simulink model "test"  (R2020a)
settings: Solver=FixedStepAuto  StartTime=0.0  StopTime=10.0  FixedStep=1e-3  RelTol=1e-3  EnableMultiTasking=on
libraries: frdmk64flib x5, etargetslib x2
settings Model: ExtModeTrigDuration=5  Creator=Windows  LastModifiedBy=Max
settings OptimizationCC: EnhancedBackFolding=on  PassReuseOutputArgsAs=Individual arguments  ZeroExternalMemoryAtStartup=off  ZeroInternalMemoryAtStartup=off  MaxStackSize=64  OptimizeBlockOrder=speed  DifferentSizesBufferReuse=on  OptimizationCustomize=off  EfficientTunableParamExpr=on
settings DebuggingCC: ParameterTunabilityLossMsg=error
settings HardwareCC: ProdBitPerPointer=32  ProdBitPerSizeT=32  ProdBitPerPtrDiffT=32  ProdLargestAtomicInteger=Long  ProdLargestAtomicFloat=Double  ProdWordSize=32  ProdHWDeviceType=ARM Compatible->ARM Cortex
settings SFSimCC: MATLABDynamicMemAlloc=off
settings RTWCC: SystemTargetFile=ert.tlc  HardwareBoard=NXP FRDM-K64F  TemplateMakefile=ert_default_tmf  Toolchain=GNU Tools for ARM Embedded Processors
settings CodeAppCC: ForceParamTrailComments=on  IgnoreCustomStorageClasses=off  OperatorAnnotations=on  SimulinkDataObjDesc=on  SFDataObjDesc=on  InsertBlockDesc=on

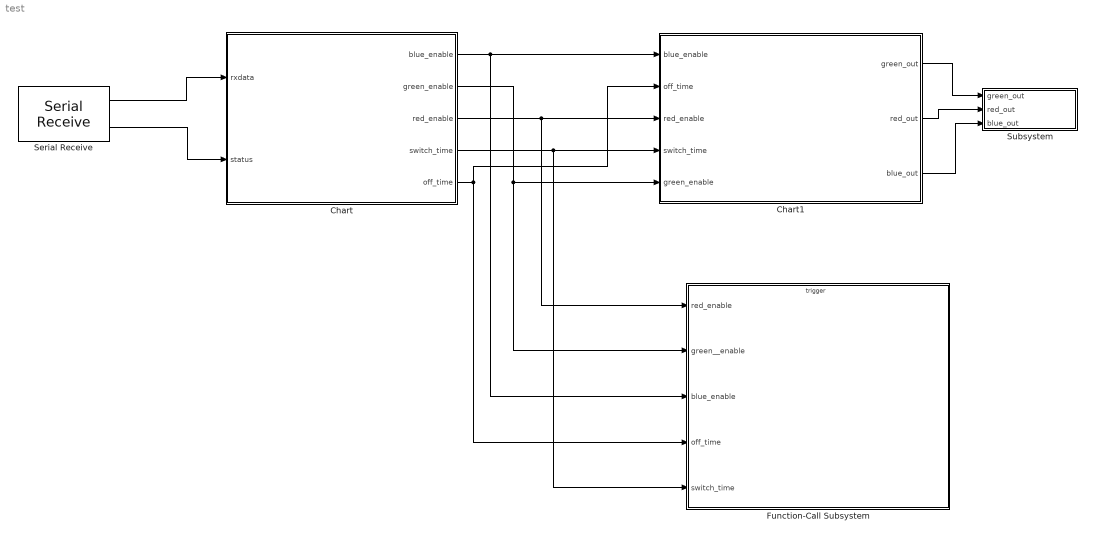
== system test ==
  Chart : Stateflow chart  TreatAsAtomicUnit=on
  Chart1 : Stateflow chart  TreatAsAtomicUnit=on
  Function-Call Subsystem : Subsystem  TreatAsAtomicUnit=on
  Serial Receive : frdmk64flib/Serial Receive  SCIModule=0  Baudrate=uint32(9600)  Parity=None  StopBits=1  HardwareFlowControl=None  ByteOrder=LittleEndian  DataType=uint8  DataLength=11  BlockingMode=off  OutputStatus=on  SampleTime=-1
  Subsystem : Subsystem
  wires:
  Serial Receive/1 -> Chart/1(rxdata)
  Serial Receive/2 -> Chart/2(status)
  Chart1/3(blue_out) -> Subsystem/3(blue_out)
  Chart/5(off_time) -> Function-Call Subsystem/4(off_time), Chart1/2(off_time)
  Chart/4(switch_time) -> Function-Call Subsystem/5(switch_time), Chart1/4(switch_time)
  Chart/3(red_enable) -> Function-Call Subsystem/1(red_enable), Chart1/3(red_enable)
  Chart/2(green_enable) -> Function-Call Subsystem/2(green__enable), Chart1/5(green_enable)
  Chart/1(blue_enable) -> Function-Call Subsystem/3(blue_enable), Chart1/1(blue_enable)
  Chart1/2(red_out) -> Subsystem/2(red_out)
  Chart1/1(green_out) -> Subsystem/1(green_out)

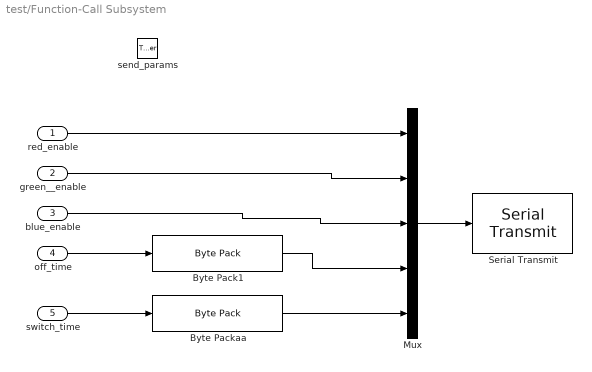
== system test/Function-Call Subsystem ==
  red_enable : Inport
  green__enable : Inport  Port=2
  blue_enable : Inport  Port=3
  off_time : Inport  Port=4
  switch_time : Inport  Port=5
  send_params : TriggerPort  TriggerType=function-call  IsSimulinkFunction=on  FunctionName=send_params  VariantControl=Variant
  Byte Pack1 : etargetslib/Byte Pack  datatypes={'single'}  byteAlign=1
  Byte Packaa : etargetslib/Byte Pack  datatypes={'uint16'}  byteAlign=1
  Mux : Mux  Inputs=5
  Serial Transmit : frdmk64flib/Serial Transmit  SCIModule=0  Baudrate=uint32(9600)  Parity=None  StopBits=1  HardwareFlowControl=None  ByteOrder=LittleEndian  BlockingMode=on  OutputStatus=off
  wires:
  red_enable/1 -> Mux/1
  switch_time/1 -> Byte Packaa/1
  off_time/1 -> Byte Pack1/1
  green__enable/1 -> Mux/2
  blue_enable/1 -> Mux/3
  Byte Pack1/1 -> Mux/4
  Byte Packaa/1 -> Mux/5
  Mux/1 -> Serial Transmit/1

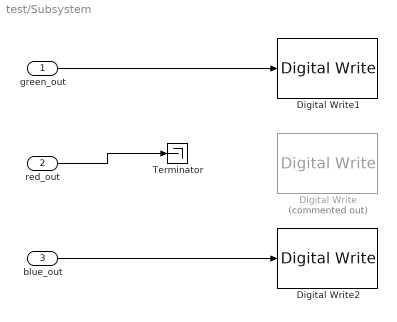
== system test/Subsystem ==
  green_out : Inport
  red_out : Inport  Port=2  OutDataTypeStr=boolean
  blue_out : Inport  Port=3
  Digital Write : frdmk64flib/Digital Write  Commented=on  Whichpin=RED_LED
  Digital Write1 : frdmk64flib/Digital Write  Whichpin=GREEN_LED
  Digital Write2 : frdmk64flib/Digital Write  Whichpin=BLUE_LED
  Terminator : Terminator
  wires:
  green_out/1 -> Digital Write1/1
  blue_out/1 -> Digital Write2/1
  red_out/1 -> Terminator/1

== stateflow chart test/Chart1 ==
  state OFF
    entry:
    red_out=false;
    green_out=false;
    blue_out=false;
  state RED_ON
    entry:
    red_out=true;
    green_out=false;
    blue_out=false;
  state BLUE_ON
    entry:
    red_out=false;
    green_out=false;
    blue_out=true;
  state GREEN_ON
    entry:
    red_out=false;
    green_out=true;
    blue_out=false;
  note: after(switch_time, msec)
  (default) -> OFF
  OFF -> (junction 3) : after(off_time, sec)
  (junction 3) -> RED_ON [order 1] : [red_enable==1]
  (junction 3) -> (junction 5) [order 2]
  RED_ON -> (junction 5) : after(switch_time,msec)
  (junction 4) -> OFF
  (junction 8) -> (junction 4) [order 2]
  (junction 5) -> (junction 8) [order 2]
  BLUE_ON -> (junction 4) : after(switch_time, msec)
  (junction 5) -> GREEN_ON [order 1] : [green_enable==1]
  (junction 8) -> BLUE_ON [order 1] : [blue_enable==1]
  GREEN_ON -> (junction 8)
  data: blue_enable input uint8; off_time input single; red_enable input uint8; switch_time input uint16; green_out output boolean; red_out output boolean; blue_out output boolean; green_enable input uint8

== stateflow chart test/Chart ==
  settings: executeAtInitialization=1
  state SET_PARAM
    entry:
    red_enable=rxdata(3);
    green_enable=rxdata(4);
    blue_enable=rxdata(5);
    off_time=typecast(rxdata(6:9), 'single');
    switch_time=typecast(rxdata(10:11), 'uint16');
  state INITIAL
    entry:
    red_enable=1;
    green_enable=1;
    blue_enable=1;
    off_time=0.5;
    switch_time=200;
  state STANDBY
  state ECHO_PARAM
    entry:
    send_params();
  SET_PARAM -> STANDBY
  (default) -> INITIAL
  (junction 13) -> SET_PARAM [order 1] : [rxdata(2)==hex2dec('55')]
  (junction 9) -> STANDBY [order 2]
  INITIAL -> STANDBY
  STANDBY -> (junction 9) : [status == 0]
  (junction 9) -> (junction 13) [order 1] : [rxdata(1)==hex2dec('16')]
  (junction 13) -> ECHO_PARAM [order 2] : [rxdata(2)==hex2dec('22')]
  ECHO_PARAM -> STANDBY
  data: rxdata input uint8; status input uint8; blue_enable output uint8; green_enable output uint8; red_enable output uint8; switch_time output uint16; off_time output single
